simulink model "pendulo_doble_sim"  (Simulink 7.2)
settings: Solver=ode4  StartTime=0.0  StopTime=20  FixedStep=0.1  RelTol=1e-3
undefined symbols (not defined in the file or in its folder): CinDirDifPendulo, CinDirPendulo2, CPDOperacional, pendulo_dobleOp, pol5G, ScalePol5G, Secuencia4p
libraries: simulink x2, roblocks x1
settings Model: Creator=dean  LastModifiedBy=dean  ExtModeAutoUpdateStatusClock=off
settings OptimizationCC: InitFltsAndDblsToZero=on
settings DebuggingCC: SaveWithParameterizedLinksMsg=none  MultiTaskDSMMsg=warning  MultiTaskCondExecSysMsg=none  StrictBusMsg=None
settings RTWCC: IncludeERTFirstTime=on

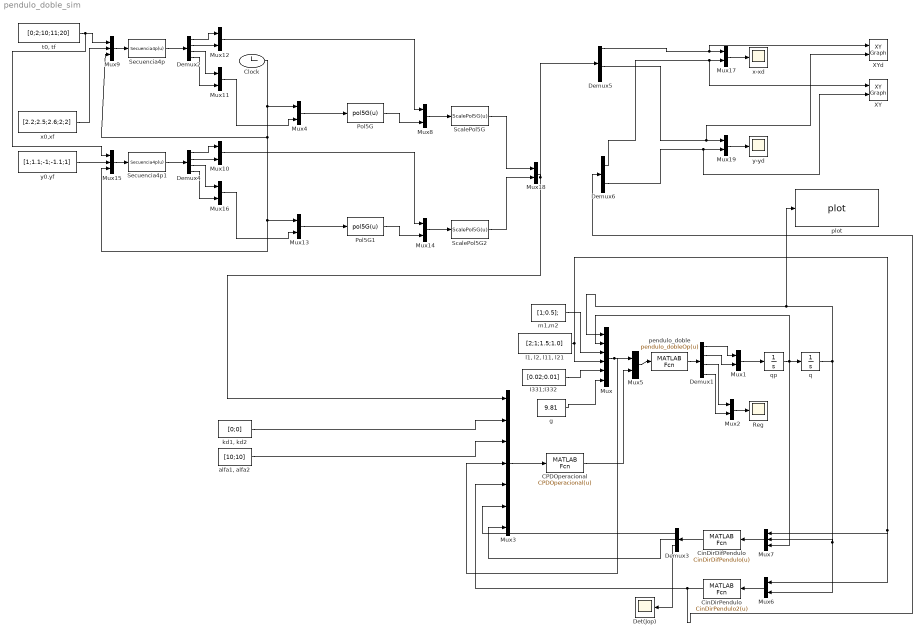
== system pendulo_doble_sim ==
  CPDOperacional : MATLABFcn  MATLABFcn=CPDOperacional(u)  OutputDimensions=2
  CinDirDifPendulo : MATLABFcn  Orientation=left  MATLABFcn=CinDirDifPendulo(u)  OutputDimensions=3
  CinDirPendulo : MATLABFcn  Orientation=left  MATLABFcn=CinDirPendulo2(u)  OutputDimensions=2
  Clock : Clock
      settings: Decimation=10
  Demux1 : Demux
  Demux2 : Demux
  Demux3 : Demux  Orientation=left  Outputs=3
  Demux4 : Demux
  Demux5 : Demux  Outputs=6
  Demux6 : Demux  Outputs=2
  Det(Jop) : Scope
      settings: TimeRange=20  YMin=1.4  YMax=2
  I331;I332 : Constant  Value=[0.02;0.01]  OutDataType=sfix(16)  OutScaling=2^0
  Mux : Mux  Inputs=6
  Mux{1..2,4..5,8,10..14,16..19} (14 alike) : Mux  Inputs=2
  Mux15 : Mux  Inputs=3
  Mux3 : Mux  Inputs=7
  Mux6 : Mux  Orientation=left  Inputs=2
  Mux7 : Mux  Orientation=left  Inputs=3
  Mux9 : Mux  Inputs=3
  Pol5G : MATLABFcn  MATLABFcn=pol5G(u)  OutputDimensions=3
  Pol5G1 : MATLABFcn  MATLABFcn=pol5G(u)  OutputDimensions=3
  Reg : Scope
      settings: YMin=-4e-015  YMax=4e-015  SaveName=ScopeData2
  ScalePol5G : MATLABFcn  MATLABFcn=ScalePol5G(u)  OutputDimensions=3
  ScalePol5G2 : MATLABFcn  MATLABFcn=ScalePol5G(u)  OutputDimensions=3
  Secuencia4p : MATLABFcn  MATLABFcn=Secuencia4p(u)  OutputDimensions=4
  Secuencia4p1 : MATLABFcn  MATLABFcn=Secuencia4p(u)  OutputDimensions=4
  XY : simulink/Sinks/XY Graph  SystemSampleTime=-1  xmin=0  xmax=3  ymin=-1.5  ymax=1.5  st=-1
  "XYd " : simulink/Sinks/XY Graph  SystemSampleTime=-1  xmin=0  xmax=3  ymin=-1.5  ymax=1.5  st=-1
  "alfa1, alfa2" : Constant  Value=[10;10]  OutDataType=sfix(16)  OutScaling=2^0
  g : Constant  Value=9.81  OutDataType=sfix(16)  OutScaling=2^0
  "kd1, kd2" : Constant  Value=[0;0]  OutDataType=sfix(16)  OutScaling=2^0
  "l1, l2, l11, l21" : Constant  Value=[2;1;1.5;1.0]  OutDataType=sfix(16)  OutScaling=2^0
  m1,m2 : Constant  Value=[1;0.5];  OutDataType=sfix(16)  OutScaling=2^0
  pendulo_doble : MATLABFcn  MATLABFcn=pendulo_dobleOp(u)  OutputDimensions=4
  plot : roblocks/plot  SystemSampleTime=-1  robot=R2GDL
  q : Integrator  InitialCondition=[0;pi/2]
  qp : Integrator  InitialCondition=[0;0]
  "t0, tf" : Constant  Value=[0;2;10;11;20]  OutDataType=sfix(16)  OutScaling=2^0
  x-xd : Scope
      settings: TimeRange=20  YMin=1.9  YMax=2.7
  x0,xf : Constant  Value=[2.2;2.5;2.6;2;2]  OutDataType=sfix(16)  OutScaling=2^0
  y-yd : Scope
      settings: TimeRange=20  YMin=0.965  YMax=1.07  SaveName=ScopeData3
  y0.yf : Constant  Value=[1;1.1;-1;-1.1;1]  OutDataType=sfix(16)  OutScaling=2^0
  wires:
  qp/1 -> q/1, Mux/2, Mux7/3
  q/1 -> Mux6/2, Mux7/2, Mux/1, plot/1
  m1,m2/1 -> Mux/3
  "l1, l2, l11, l21"/1 -> Mux/4, Mux6/1, Mux7/1
  I331;I332/1 -> Mux/5
  g/1 -> Mux/6
  pendulo_doble/1 -> Demux1/1
  Demux1/1 -> Mux1/1
  Demux1/2 -> Mux1/2
  Mux1/1 -> qp/1
  Demux1/3 -> Mux2/1
  Demux1/4 -> Mux2/2
  Mux2/1 -> Reg/1
  Mux3/1 -> CPDOperacional/1
  "kd1, kd2"/1 -> Mux3/2
  "alfa1, alfa2"/1 -> Mux3/3
  Mux4/1 -> Pol5G/1
  Clock/1 -> Mux4/1, Mux9/3, Mux13/1, Mux15/3
  Mux8/1 -> ScalePol5G/1
  Pol5G/1 -> Mux8/2
  Mux9/1 -> Secuencia4p/1
  "t0, tf"/1 -> Mux9/1, Mux15/1
  x0,xf/1 -> Mux9/2
  Secuencia4p/1 -> Demux2/1
  Demux2/1 -> Mux12/1
  Demux2/2 -> Mux12/2
  Demux2/3 -> Mux11/1
  Demux2/4 -> Mux11/2
  Mux11/1 -> Mux4/2
  Mux12/1 -> Mux8/1
  Mux13/1 -> Pol5G1/1
  Mux14/1 -> ScalePol5G2/1
  Pol5G1/1 -> Mux14/2
  Mux15/1 -> Secuencia4p1/1
  y0.yf/1 -> Mux15/2
  Secuencia4p1/1 -> Demux4/1
  Demux4/1 -> Mux10/1
  Demux4/2 -> Mux10/2
  Demux4/3 -> Mux16/1
  Demux4/4 -> Mux16/2
  Mux16/1 -> Mux13/2
  Mux10/1 -> Mux14/1
  ScalePol5G/1 -> Mux18/1
  ScalePol5G2/1 -> Mux18/2
  Mux18/1 -> Mux3/1, Demux5/1
  Mux5/1 -> pendulo_doble/1
  Mux/1 -> Mux5/1, Mux3/4
  CinDirPendulo/1 -> Mux3/5, Demux6/1
  Mux6/1 -> CinDirPendulo/1
  Mux7/1 -> CinDirDifPendulo/1
  CinDirDifPendulo/1 -> Demux3/1
  Demux3/1 -> Mux3/6
  Demux3/2 -> Mux3/7
  Demux3/3 -> Det(Jop)/1
  CPDOperacional/1 -> Mux5/2
  Mux17/1 -> x-xd/1
  Demux5/1 -> Mux17/1, "XYd "/1
  Mux19/1 -> y-yd/1
  Demux5/4 -> Mux19/1, "XYd "/2
  Demux6/1 -> Mux17/2, XY/1
  Demux6/2 -> Mux19/2, XY/2
